simulink model "B42"  (R2015a)
settings: Solver=ode45  StartTime=0.0  StopTime=10.0  RelTol=1e-3
libraries: commchan3 x1, commsink2 x1, commutil2 x1, commfilt2 x1, commrandsrc2 x1, dspstat3 x1
settings Model: Creator=Ekko  LastModifiedBy=Ekko

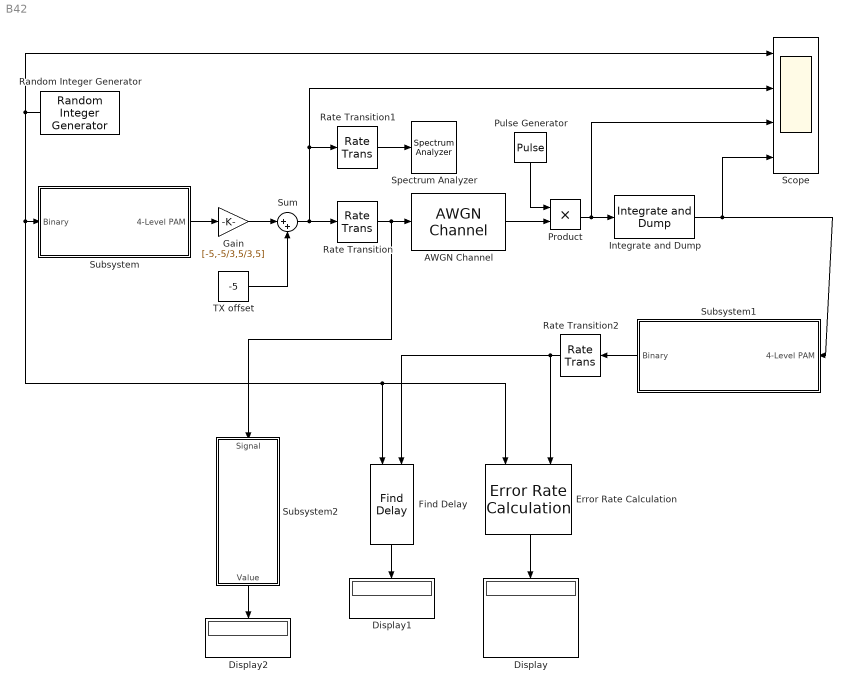
== system B42 ==
  AWGN Channel : commchan3/AWGN Channel  InputProcessing=Columns as channels (frame based)  seed=67  noiseMode="Signal to noise ratio  (Eb/No)"  EbNodB=10  EsNodB=10  SNRdB=10  bitsPerSym=1  Ps=1  Tsym=1e-5  variance=1
  Display : Display
  Display1 : Display
  Display2 : Display
  Error Rate Calculation : commsink2/Error Rate Calculation  N=0  st_delay=0  cp_mode=Entire frame  subframe=[]  PMode=Port  WsName=ErrorVec  RsMode2=off  stop=off  numErr=100  maxBits=1e6
  Find Delay : commutil2/Find Delay  corrLength=200  chgSigOP=off  stopUpdate=off  numConstDelay=3
  Gain : Gain  Gain=[-5,-5/3,5/3,5]
  Integrate and Dump : commfilt2/Integrate and Dump  obssamples=4  offsetsamples=0  nodump=off  roundingMode=Floor  overflowMode=off
  Product : Product
  Pulse Generator : DiscretePulseGenerator  Amplitude=2  Period=10  PulseWidth=5  SampleTime=2e-5
  Random Integer Generator : commrandsrc2/Random Integer Generator  mul=2  seed=37  Ts=1e-5  frameBased=off  sampPerFrame=1  orient=off  outDataType=double
  Rate Transition : RateTransition  Deterministic=off  OutPortSampleTime=1e-5
  Rate Transition1 : RateTransition  Deterministic=off  OutPortSampleTime=1e-5
  Rate Transition2 : RateTransition  Deterministic=off  OutPortSampleTime=1e-5
  Scope : Scope  NumInputPorts=4
      settings: YMin=-5~-5~-5~-5  YMax=5~5~5~5
  Spectrum Analyzer : SpectrumAnalyzer
  Subsystem : Subsystem
  Subsystem1 : Subsystem
  Subsystem2 : Subsystem
  Sum : Sum  Inputs=|++
  "TX offset " : Constant  Value=-5  SampleTime=1e-6
  wires:
  Subsystem/1(4-Level PAM) -> Gain/1
  Gain/1 -> Sum/1
  "TX offset "/1 -> Sum/2
  Sum/1 -> Scope/2, Rate Transition1/1, Rate Transition/1
  Rate Transition1/1 -> Spectrum Analyzer/1
  Rate Transition/1 -> Subsystem2/1("Signal "), AWGN Channel/1
  Random Integer Generator/1 -> Find Delay/1, Error Rate Calculation/1, Subsystem/1("Binary "), Scope/1
  Pulse Generator/1 -> Product/1
  AWGN Channel/1 -> Product/2
  Subsystem2/1("Value ") -> Display2/1
  Find Delay/1 -> Display1/1
  Rate Transition2/1 -> Find Delay/2, Error Rate Calculation/2
  Error Rate Calculation/1 -> Display/1
  Subsystem1/1("Binary ") -> Rate Transition2/1
  Product/1 -> Scope/3, Integrate and Dump/1
  Integrate and Dump/1 -> Scope/4, Subsystem1/1("4-Level PAM ")

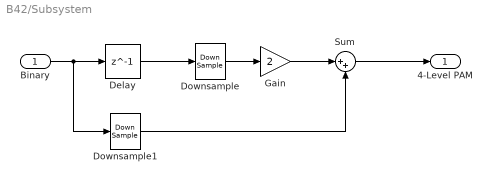
== system B42/Subsystem ==
  "Binary " : Inport
  Delay : Delay  DelayLength=1
  Downsample : DownSample  RateOptions=Allow multirate processing
  Downsample1 : DownSample  RateOptions=Allow multirate processing
  Gain : Gain  Gain=2
  Sum : Sum  Inputs=|++
  4-Level PAM : Outport
  wires:
  Gain/1 -> Sum/1
  Downsample1/1 -> Sum/2
  Sum/1 -> 4-Level PAM/1
  Delay/1 -> Downsample/1
  Downsample/1 -> Gain/1
  "Binary "/1 -> Downsample1/1, Delay/1

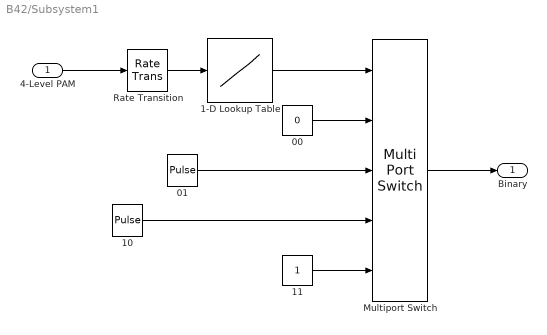
== system B42/Subsystem1 ==
  "4-Level PAM " : Inport
  00 : Constant  Value=0  SampleTime=2e-5
  "01 " : DiscretePulseGenerator  Amplitude=2  Period=50  PulseWidth=5  SampleTime=1e-5
  1-D Lookup Table : Lookup_n-D  NumberOfTableDimensions=1  BreakpointsForDimension1=[-5:5]  Table=tanh([-5:5])  InternalRulePriority=Speed  RndMeth=Simplest  InputSameDT=on
  10 : DiscretePulseGenerator  Amplitude=2  Period=10  PulseWidth=5  SampleTime=1e-5
  "11 " : Constant  SampleTime=2e-5
  Multiport Switch : MultiPortSwitch  Inputs=4  DiagnosticForDefault=None
  Rate Transition : RateTransition  Deterministic=off  X0=1e3  OutPortSampleTime=1e-5
  "Binary " : Outport
  wires:
  Rate Transition/1 -> 1-D Lookup Table/1
  "4-Level PAM "/1 -> Rate Transition/1
  1-D Lookup Table/1 -> Multiport Switch/1
  "11 "/1 -> Multiport Switch/5
  10/1 -> Multiport Switch/4
  Multiport Switch/1 -> "Binary "/1
  "01 "/1 -> Multiport Switch/3
  00/1 -> Multiport Switch/2

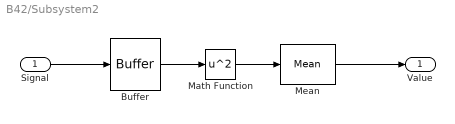
== system B42/Subsystem2 ==
  "Signal " : Inport
  Buffer : Buffer  TreatMby1Signals=One channel
  Math Function : Math  Operator=square  SaturateOnIntegerOverflow=on
  Mean : dspstat3/Mean  run=off  reset_popup=None  InputProcessing=Columns as channels (frame based)  directionMode=Each column  dimension=1  treatSBRowAsCol=off  roiEnable=off  roiType=Rectangles  roiPortion=Entire ROI  roiOutput=Individual statistics for each ROI  roiFlag=off  outputDataTypeStr=Inherit: Same as accumulator  outputLastDataTypeStr=Inherit: Same as accumulator  outputMin=[]  outputMax=[]  roundingMode=Floor  overflowMode=off
  "Value " : Outport
  wires:
  "Signal "/1 -> Buffer/1
  Mean/1 -> "Value "/1
  Math Function/1 -> Mean/1
  Buffer/1 -> Math Function/1
